simulink model "pendule_inv_etu"  (R2021a)
settings: Solver=VariableStepAuto  StartTime=0.0  StopTime=10.0  RelTol=1e-3
values from neighbouring files (symbols this model uses):
  g = 9.81    [simu_pendule_inv_capteur_etu.m]    (also in simu_pendule_inv_echant_etu.m; simu_pendule_inv_etu.m)
  K = [10 1]    [simu_pendule_inv_capteur_etu.m]    (also in simu_pendule_inv_echant_etu.m = [30 10]; simu_pendule_inv_etu.m = [30 10])
  l = 10    [simu_pendule_inv_capteur_etu.m]    (also in simu_pendule_inv_echant_etu.m; simu_pendule_inv_etu.m)
  ue = 0    [simu_pendule_inv_capteur_etu.m]    (also in simu_pendule_inv_echant_etu.m; simu_pendule_inv_etu.m)
  x0 = [pi/20 0]'    [simu_pendule_inv_capteur_etu.m]    (also in simu_pendule_inv_echant_etu.m; simu_pendule_inv_etu.m = [pi/10 0]')
  xe = [0 0]'    [simu_pendule_inv_capteur_etu.m]    (also in simu_pendule_inv_echant_etu.m; simu_pendule_inv_etu.m)
settings Model: Creator=cdelmair  LastModifiedBy=cdelmair

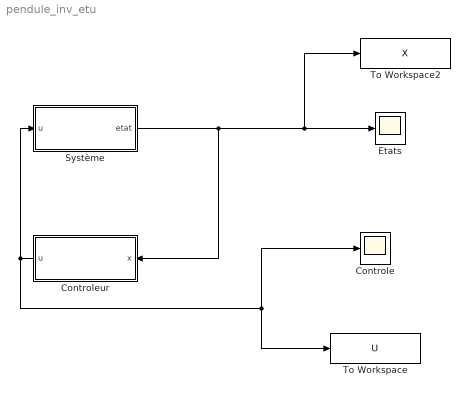
== system pendule_inv_etu ==
  Controle : Scope
  Controleur : Subsystem
  Etats : Scope
  Système : Subsystem
  To Workspace : ToWorkspace  VariableName=U  SaveFormat=Timeseries  SampleTime=-1
  To Workspace2 : ToWorkspace  VariableName=X  SaveFormat=Timeseries  SampleTime=-1
  wires:
  Controleur/1(u) -> To Workspace/1, Controle/1, Système/1(u)
  Système/1(etat) -> Controleur/1(x), To Workspace2/1, Etats/1

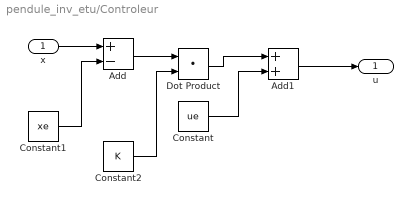
== system pendule_inv_etu/Controleur ==
  x : Inport
  Add : Sum  Inputs=+-
  Add1 : Sum
  Constant : Constant  Value=ue
  Constant1 : Constant  Value=xe
  Constant2 : Constant  Value=K
  Dot Product : DotProduct  InputSameDT=on  OutDataTypeStr=Inherit: Inherit via internal rule
  u : Outport
  wires:
  x/1 -> Add/1
  Constant1/1 -> Add/2
  Constant/1 -> Add1/2
  Add1/1 -> u/1
  Dot Product/1 -> Add1/1
  Add/1 -> Dot Product/1
  Constant2/1 -> Dot Product/2

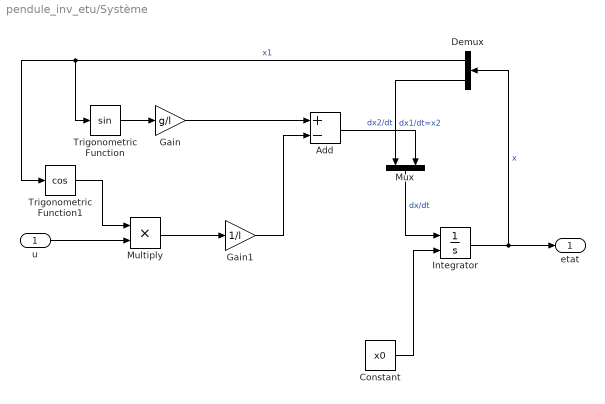
== system pendule_inv_etu/Système ==
  u : Inport
  Add : Sum  Inputs=+-
  Constant : Constant  Value=x0
  Demux : Demux  Outputs=2
  Gain : Gain  Gain=g/l
  Gain1 : Gain  Gain=1/l
  Integrator : Integrator  InitialConditionSource=external
  Multiply : Product  Inputs=**
  Mux : Mux  Inputs=2
  Trigonometric Function : Trigonometry
  Trigonometric Function1 : Trigonometry  Operator=cos
  etat : Outport
  wires:
  Trigonometric Function/1 -> Gain/1
  Gain/1 -> Add/1
  u/1 -> Multiply/2
  Trigonometric Function1/1 -> Multiply/1
  Multiply/1 -> Gain1/1
  Gain1/1 -> Add/2
  Integrator/1 -> Demux/1, etat/1  "x"
  Constant/1 -> Integrator/2
  Demux/1 -> Trigonometric Function1/1, Trigonometric Function/1  "x1"
  Demux/2 -> Mux/1  "dx1/dt=x2"
  Add/1 -> Mux/2  "dx2/dt"
  Mux/1 -> Integrator/1  "dx/dt"
